simulink model "ACC_Controller"  (R2025b)
settings: Solver=ode4  StartTime=0.0  StopTime=30  FixedStep=0.01  RelTol=1e-3
libraries: simulink x1
settings Model: Creator=ghazal  LastModifiedBy=ghazal

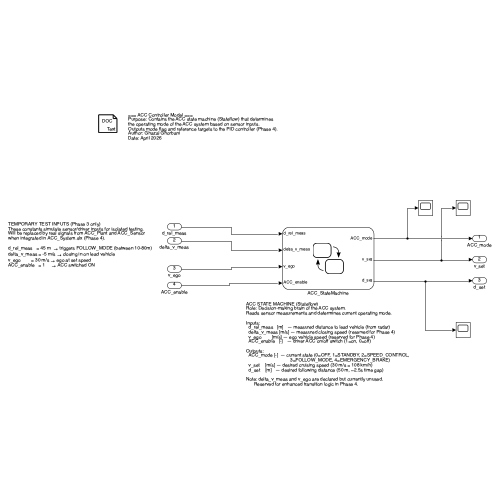
[thumbnail: Simulink's stored preview of the top-level diagram]
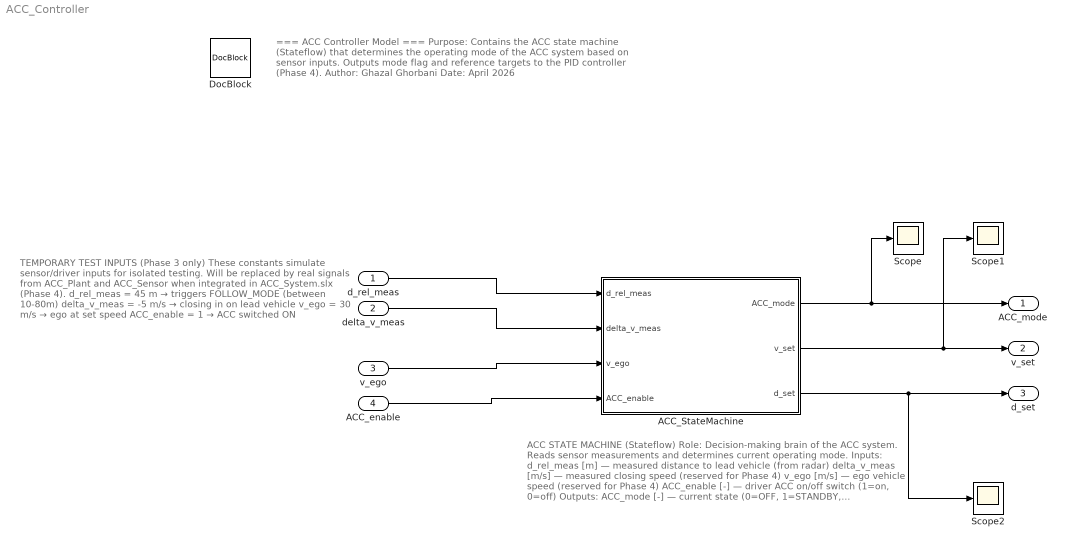
== system ACC_Controller ==
  note: TEMPORARY TEST INPUTS (Phase 3 only)
      | These constants simulate sensor/driver inputs for isolated testing.
      | Will be replaced by real signals from ACC_Plant and ACC_Sensor
      | when integrated in ACC_System.slx (Phase 4).
      |
      | d_rel_meas   = 45 m  → triggers FOLLOW_MODE (between 10-80m)
      | delta_v_meas = -5 m/s → closing in on lead vehicle
      | v_ego        = 30 m/s → ego at set speed
      | ACC_enable   = 1     → ACC switched ON
  note: ACC STATE MACHINE (Stateflow)
      | Role: Decision-making brain of the ACC system.
      | Reads sensor measurements and determines current operating mode.
      |
      | Inputs:
      |   d_rel_meas   [m]   — measured distance to lead vehicle (from radar)
      |   delta_v_meas [m/s] — measured closing speed (reserved for Phase 4)
      |   v_ego        [m/s] — ego vehicle speed (reserved for Phase 4)
      |   ACC_enable   [-]   — driver ACC on/off switch (1=on, 0=off)
      |
      | Outputs:
      |   ACC_mode [-]  — current state (0=OFF, 1=STANDBY, 2=SPEED_CONTROL,
      |                                   3=FOLLOW_MODE, 4=EMERGENCY_BRAKE)
      |   v_set    [m/s] — desired cruising speed (30 m/s = 108 km/h)
      |   d_set    [m]   — desired following distance (50 m, ~2.5s time gap)
      |
      | Note: delta_v_meas and v_ego are declared but currently unused.
      |       Reserved for enhanced transition logic in Phase 4.
  note: === ACC Controller Model ===
      | Purpose: Contains the ACC state machine (Stateflow) that determines
      | the operating mode of the ACC system based on sensor inputs.
      | Outputs mode flag and reference targets to the PID controller (Phase 4).
      | Author: Ghazal Ghorbani
      | Date: April 2026
  d_rel_meas : Inport
  delta_v_meas : Inport  Port=2
  v_ego : Inport  Port=3
  ACC_enable : Inport  Port=4
  ACC_StateMachine : Stateflow chart  TreatAsAtomicUnit=on
  DocBlock : simulink/Model-Wide Utilities/DocBlock  DocumentType=Text
      content=|
      | STATEFLOW CHART: ACC_StateMachine
      | ========================================
      | DESCRIPTION:
      |   Hierarchical state machine implementing the operating mode logic
      |   for an Adaptive Cruise Control system. Determines which control
      |   law the PID controller (Phase 4) should apply at each instant.
      |
      | STATES:
      |   OFF (default)
      |     Condition : ACC_enable == 0
      |     Behaviour : System inactive. All outputs zeroed.
      |     ACC_mode  : 0
      |
      |   STANDBY
      |     Condition : ACC_enable == 1, no clear road/lead condition yet
      |     Behaviour : ACC enabled and waiting. Ready to transition.
      |     ACC_mode  : 1
      |
      |   SPEED_CONTROL
      |     Condition : d_rel_meas > 80m (road clear ahead)
      |     Behaviour : Maintain set speed v_set = 30 m/s.
      |                 PID controls v_ego → v_set.
      |     ACC_mode  : 2
      |
      |   FOLLOW_MODE
      |     Condition : 10m < d_rel_meas <= 80m (lead vehicle detected)
      |     Behaviour : Maintain safe following distance d_set = 50m.
      |                 PID controls d_rel → d_set.
      |                 Speed naturally drops below v_set to match lead.
      |     ACC_mode  : 3
      |
      |   EMERGENCY_BRAKE
      |     Condition : d_rel_meas <= 10m (critically close)
      |     Behaviour : Maximum braking commanded.
      |                 v_set set to 0 to force full deceleration.
      |     ACC_mode  : 4
      |
      | TRANSITIONS (priority order):
      |   OFF           → STANDBY        : [ACC_enable == 1]
      |   STANDBY       → OFF            : [ACC_enable == 0]
      |   STANDBY       → SPEED_CONTROL  : [d_rel_meas > 80]
      |   STANDBY       → FOLLOW_MODE    : [d_rel_meas <= 80 && d_rel_meas > 10]
      |   SPEED_CONTROL → STANDBY        : [ACC_enable == 0]
      |   SPEED_CONTROL → FOLLOW_MODE    : [d_rel_meas <= 80 && d_rel_meas > 10]
      |   FOLLOW_MODE   → SPEED_CONTROL  : [d_rel_meas > 80]
      |   FOLLOW_MODE   → EMERGENCY_BRAKE: [d_rel_meas <= 10]
      |   EMERGENCY_BRAKE → FOLLOW_MODE  : [d_rel_meas > 10 && d_rel_meas <= 80]
      |   EMERGENCY_BRAKE → STANDBY      : [ACC_enable == 0]
      |
      | DESIGN PARAMETERS:
      |   v_set = 30 m/s (108 km/h)
      |     Rationale: Realistic European highway cruising speed.
      |                Faster than both ego (20 m/s) and lead (15 m/s)
      |                to create meaningful control behaviour.
      |
      |   d_set = 50 m
      |     Rationale: Based on ISO 15622 time-gap law:
      |                d_set = d_standstill + t_gap × v_ego
      |                d_set = 5 + 2.5 × 18 ≈ 50 m
      |                (2.5s time gap — ISO recommended value)
      |
      | DISTANCE THRESHOLDS:
      |   > 80m  : Road considered clear → SPEED_CONTROL
      |   10–80m : Lead vehicle in range → FOLLOW_MODE
      |   <= 10m : Critical distance     → EMERGENCY_BRAKE
      |     Rationale: At ego speed ~20 m/s, 10m = 0.5s reaction distance.
      |                Below this, only emergency braking can prevent collision.
      |
      | UNUSED INPUTS (reserved for Phase 4):
      |   delta_v_meas : Will be used for combined distance+velocity
      |                  transition conditions (e.g. fast closing at medium range)
      |   v_ego        : Will be used for dynamic d_set calculation and
      |                  speed error computation in PID controller
      |
      | VALIDATION:
      |   Test with d_rel_meas=45, ACC_enable=1:
      |   Expected ACC_mode sequence: 0 → 1 → 3 (OFF→STANDBY→FOLLOW_MODE)
  Scope : Scope
      settings: ActiveDisplayYMinimum=-0.37499999999999989  ActiveDisplayYMaximum=3.375
  Scope1 : Scope
      settings: ActiveDisplayYMinimum=-3.7499999999999991  ActiveDisplayYMaximum=33.75
  Scope2 : Scope
      settings: ActiveDisplayYMinimum=-6.2499999999999982  ActiveDisplayYMaximum=56.25  DataLoggingVariableName=ScopeData2
  ACC_mode : Outport
  v_set : Outport  Port=2
  d_set : Outport  Port=3
  wires:
  ACC_StateMachine/1(ACC_mode) -> Scope/1, ACC_mode/1
  ACC_StateMachine/2(v_set) -> Scope1/1, v_set/1
  ACC_StateMachine/3(d_set) -> Scope2/1, d_set/1
  d_rel_meas/1 -> ACC_StateMachine/1(d_rel_meas)
  delta_v_meas/1 -> ACC_StateMachine/2(delta_v_meas)
  v_ego/1 -> ACC_StateMachine/3(v_ego)
  ACC_enable/1 -> ACC_StateMachine/4(ACC_enable)

== stateflow chart ACC_Controller/ACC_StateMachine ==
  note: === ACC State Machine Documentation ===
      | Purpose: Determines ACC operating mode based on sensor inputs.
      |
      | STATES & ACC_mode values:
      |   OFF              (0) — ACC disabled by driver
      |   STANDBY          (1) — ACC enabled, waiting
      |   SPEED_CONTROL    (2) — Road clear, maintaining v_set=30 m/s
      |   FOLLOW_MODE      (3) — Lead detected, maintaining d_set=50 m
      |   EMERGENCY_BRAKE  (4) — Critical distance <=10m, max braking
      |
      | DISTANCE THRESHOLDS:
      |   d_rel > 80m      → SPEED_CONTROL
      |   10m < d_rel <= 80m → FOLLOW_MODE
      |   d_rel <= 10m     → EMERGENCY_BRAKE
      |
      | UNUSED INPUTS (reserved for Phase 4):
      |   delta_v_meas, v_ego — will be used in PID controller
  state OFF
    entry:
    ACC_mode = 0;
    v_set = 0;
    d_set = 0;
    settings: description=|
        | Default state. System inactive at startup or when driver
        | disables ACC. All outputs zeroed. ACC_mode = 0.
  state STANDBY
    entry:
    ACC_mode = 1;
    v_set = 30;
    d_set = 50;
    settings: description=|
        | ACC enabled. Waiting for road condition to be assessed.
        | Transitions to SPEED_CONTROL if road clear (>80m),
        | or FOLLOW_MODE if lead vehicle detected (10-80m).
        | ACC_mode = 1.
  state SPEED_CONTROL
    entry:
    ACC_mode = 2;
    v_set = 30;
    d_set = 50;
    settings: description=|
        | No lead vehicle within 80m. PID controller regulates
        | ego speed toward v_set = 30 m/s (108 km/h).
        | ACC_mode = 2.
  state EMERGENCY_BRAKE
    entry:
    ACC_mode = 4;
    v_set = 0;
    d_set = 50;
    settings: description=|
        | Critical distance <= 10m. Maximum braking commanded.
        | At 20 m/s, 10m = 0.5s to collision — human reaction
        | time is ~1.5s, so automated emergency braking essential.
        | ACC_mode = 4.
  state FOLLOW_MODE
    entry:
    ACC_mode = 3;
    v_set = 30;
    d_set = 50;
    settings: description=|
        | Lead vehicle detected between 10-80m. PID controller
        | regulates gap toward d_set = 50m (ISO 15622 time-gap law,
        | 2.5s at ~18 m/s). Speed naturally drops below v_set.
        | ACC_mode = 3.
  EMERGENCY_BRAKE -> STANDBY [order 2] : [ACC_enable == 0]
  (default) -> OFF
  STANDBY -> SPEED_CONTROL [order 2] : [d_rel_meas > 80]
  OFF -> STANDBY : [ACC_enable == 1]
  SPEED_CONTROL -> STANDBY [order 1] : [ACC_enable == 0]
  STANDBY -> OFF [order 1] : [ACC_enable == 0]
  STANDBY -> FOLLOW_MODE [order 3] : [d_rel_meas <= 80 && d_rel_meas > 10]
  SPEED_CONTROL -> FOLLOW_MODE [order 2] : [d_rel_meas <= 80 && d_rel_meas > 10]
  FOLLOW_MODE -> SPEED_CONTROL [order 1] : [d_rel_meas > 80]
  EMERGENCY_BRAKE -> FOLLOW_MODE [order 1] : [d_rel_meas > 10 && d_rel_meas <= 80]
  FOLLOW_MODE -> EMERGENCY_BRAKE [order 2] : [d_rel_meas <= 10]
  data: d_rel_meas input; delta_v_meas input; v_ego input; ACC_enable input; ACC_mode output; v_set output; d_set output
